simulink model "CCToACCFinal1"  (R2025b)
settings: Solver=VariableStepAuto  StartTime=0.0  StopTime=40  RelTol=1e-3
undefined symbols (not defined in the file or in its folder): Cd_air, Cr, default_spacing, m, Sim3dSensor, theta, time_gap, v_set
libraries: drivingscenarioandsensors x5, sim3dautolib x2, sim3dcameralib x1, sim3dlib x1, simulink x1
(part 1 of 4)
settings Model: Creator=Harshal  LastModifiedBy=PARSYSTEM

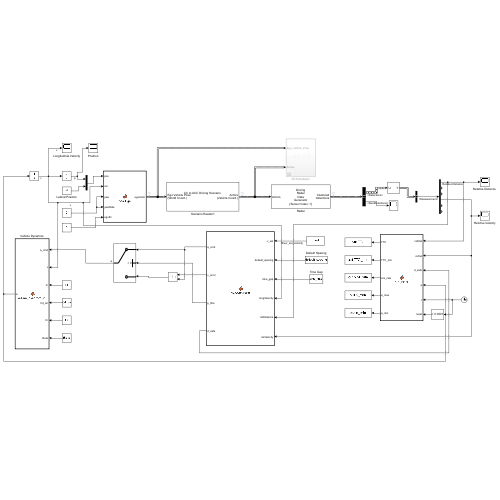
[thumbnail: Simulink's stored preview of the top-level diagram]
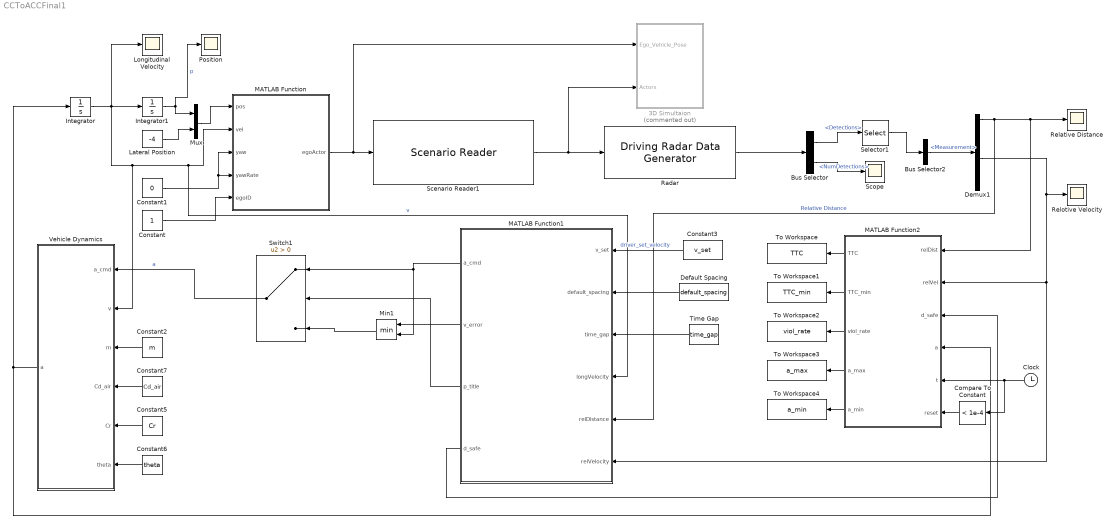
== system CCToACCFinal1 ==
  3D Simultaion : Subsystem  Commented=on
  Bus Selector : BusSelector  OutputSignals=Detections,NumDetections
  Bus Selector2 : BusSelector  OutputSignals=Measurement
  Clock : Clock
  Compare To Constant : simulink/Logic and Bit Operations/Compare To Constant  relop=<  const=1e-4  OutDataTypeStr=boolean
  Constant : Constant
  Constant1 : Constant  Value=0
  Constant2 : Constant  Value=m
  Constant3 : Constant  Value=v_set
  Constant5 : Constant  Value=Cr
  Constant6 : Constant  Value=theta
  Constant7 : Constant  Value=Cd_air
  Default Spacing : Constant  Value=default_spacing  SampleTime=0
  Demux1 : Demux  Outputs=6
  Integrator : Integrator
  Integrator1 : Integrator
  Lateral Position : Constant  Value=-4
  Longitudinal Velocity : Scope
      settings: ActiveDisplayYMinimum=-1.50449  ActiveDisplayYMaximum=13.5404  DataLoggingVariableName=ScopeData6
  MATLAB Function : MATLAB Function  TreatAsAtomicUnit=on
  MATLAB Function1 : MATLAB Function  TreatAsAtomicUnit=on
  MATLAB Function2 : MATLAB Function  TreatAsAtomicUnit=on
  Min1 : MinMax  Inputs=2
  Mux : Mux  Inputs=2
  Position : Scope
      settings: ActiveDisplayYMinimum=-48.19824  ActiveDisplayYMaximum=433.78413  DataLoggingVariableName=ScopeData3
